simulink model "WaterTank_system"  (R2024b)
settings: Solver=VariableStepAuto  StartTime=0.0  StopTime=200  RelTol=1e-3
libraries: simulink x2, rllib x1
settings Model: Creator=ROG  LastModifiedBy=DELL

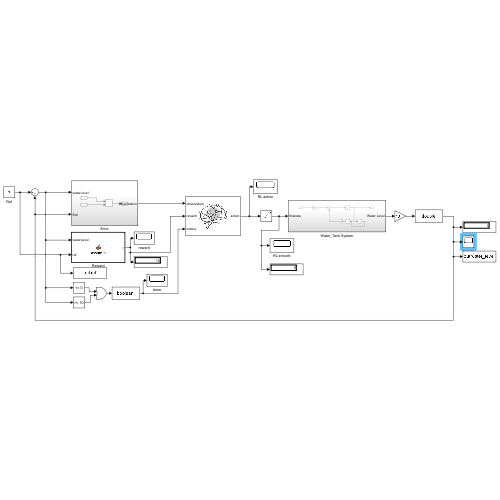
[thumbnail: Simulink's stored preview of the top-level diagram]
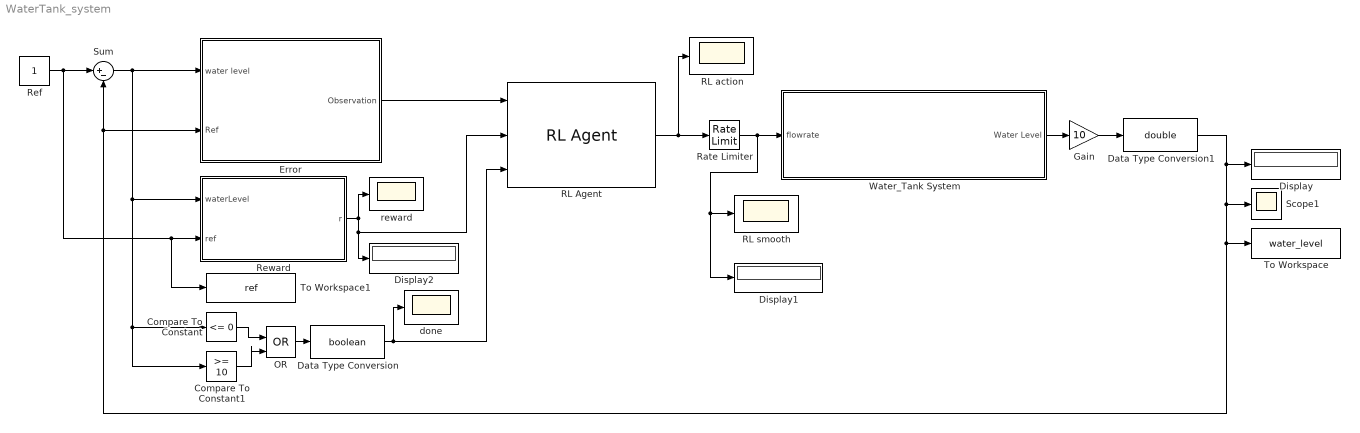
== system WaterTank_system ==
  Compare To Constant : simulink/Logic and Bit Operations/Compare To Constant  relop=<=  const=0  OutDataTypeStr=boolean
  Compare To Constant1 : simulink/Logic and Bit Operations/Compare To Constant  relop=>=  const=10  OutDataTypeStr=boolean
  Data Type Conversion : DataTypeConversion  OutDataTypeStr=boolean  SaturateOnIntegerOverflow=off  RndMeth=Floor
  Data Type Conversion1 : DataTypeConversion  OutDataTypeStr=double  SaturateOnIntegerOverflow=off  RndMeth=Floor
  Display : Display
  Display1 : Display
  Display2 : Display
  Error : Subsystem
  Gain : Gain  Gain=10
  OR : Logic  Operator=OR  IconShape=distinctive  AllPortsSameDT=off  OutDataTypeStr=boolean
  RL Agent : rllib/RL Agent  Agent=agent  ExternalActionAsInput=off  ProvideLastAction=off  ProvideCumRwd=off  TreatAsDirectFeedthrough=on  UseStrictObservationDataTypes=off
  RL action : Scope
  RL smooth : Scope
  Rate Limiter : RateLimiter
  Ref : Constant
  Reward : MATLAB Function  TreatAsAtomicUnit=on
  Scope1 : Scope
  Sum : Sum  Inputs=|+-
  To Workspace : ToWorkspace  VariableName=water_level  SaveFormat=Structure With Time  SampleTime=-1
  To Workspace1 : ToWorkspace  VariableName=ref  SaveFormat=Structure With Time  SampleTime=-1
  Water_Tank System : Subsystem
  done : Scope
  reward : Scope
  wires:
  Ref/1 -> To Workspace1/1, Reward/2(ref), Sum/1
  Sum/1 -> Error/1(water level), Compare To Constant1/1, Compare To Constant/1, Reward/1(waterLevel)
  Reward/1(r) -> Display2/1, RL Agent/2, reward/1
  Error/1(Observation) -> RL Agent/1
  Water_Tank System/1(Water Level) -> Gain/1
  RL Agent/1 -> RL action/1, Rate Limiter/1
  Compare To Constant/1 -> OR/1
  Compare To Constant1/1 -> OR/2
  OR/1 -> Data Type Conversion/1
  Data Type Conversion/1 -> RL Agent/3, done/1
  Rate Limiter/1 -> Display1/1, RL smooth/1, Water_Tank System/1(flowrate)
  Gain/1 -> Data Type Conversion1/1
  Data Type Conversion1/1 -> To Workspace/1, Error/2(Ref), Sum/2, Scope1/1, Display/1

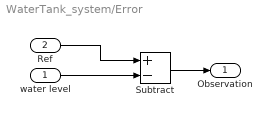
== system WaterTank_system/Error ==
  water level : Inport
  Ref : Inport  Port=2
  Subtract : Sum  Inputs=+-
  Observation : Outport
  wires:
  Ref/1 -> Subtract/1
  water level/1 -> Subtract/2
  Subtract/1 -> Observation/1

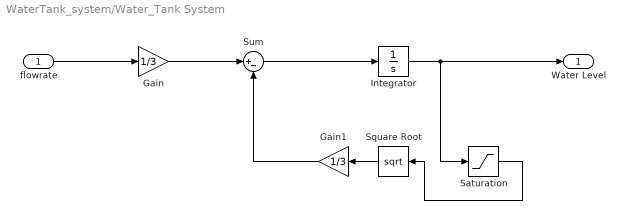
== system WaterTank_system/Water_Tank System ==
  flowrate : Inport
  Gain : Gain  Gain=1/3
  Gain1 : Gain  Gain=1/3
  Integrator : Integrator
  Saturation : Saturate  UpperLimit=inf  LowerLimit=0
  Square Root : Sqrt  OutputSignalType=real
  Sum : Sum  Inputs=|+-  OutDataTypeStr=Inherit: Same as first input
  Water Level : Outport
  wires:
  flowrate/1 -> Gain/1
  Sum/1 -> Integrator/1
  Gain1/1 -> Sum/2
  Gain/1 -> Sum/1
  Square Root/1 -> Gain1/1
  Integrator/1 -> Saturation/1, Water Level/1
  Saturation/1 -> Square Root/1

== matlab function WaterTank_system/Reward ==
  data: waterLevel input; r output; ref input
function r = RewardFn(waterLevel,ref)
    error = abs(waterLevel - ref);
    
    if error < 0.05
        r = 10;  % Perfectly near target
    else
        r = -error;  % Penalize based on distance
    end
end
